simulink model "Super3"  (Simulink 5.0)
settings: Solver=ode45  StartTime=0.0  StopTime=10.0  RelTol=1e-3
undefined symbols (not defined in the file): sigbuilder_block
settings Model: Creator=scaife  LastModifiedBy=scaife  ExtModeAutoUpdateStatusClock=off

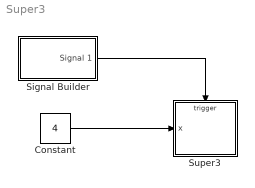
== system Super3 ==
  Constant : Constant  Value=4
  Signal Builder : Subsystem  Tag=STV Subsys  StartFcn=sigbuilder_block('start');  StopFcn=sigbuilder_block('stop');  ClipboardFcn=sigbuilder_block('clipboard');  mask(Sigbuilder block){}
      mask help: Sigbuilder GUI
      mask init:
      | if ~strcmp(get_param(bdroot(gcb),'SimulationStatus'),'stopped') tuvar = sigbuilder_block('maskInit'); end
      settings: CopyFcn=sigbuilder_block('copy');  DeleteFcn=sigbuilder_block('delete');  ModelCloseFcn=sigbuilder_block('modelClose');  PreSaveFcn=sigbuilder_block('preSave');  NameChangeFcn=sigbuilder_block('namechange');  OpenFcn=sigbuilder_block('open',[50 50 520 400 ]);  CloseFcn=sigbuilder_block('close');
      mask Display: plot(0,0,100,100,[10,10,40,40,10],[80,20,20,80,80],[40,10],[50,50], [40,27,10],[65,72,56],[40,25,25,10],[28,28,43,43]);
  Super3 : Stateflow chart
  wires:
  Signal Builder/1(Signal 1) -> Super3/Trigger
  Constant/1 -> Super3/1(x)

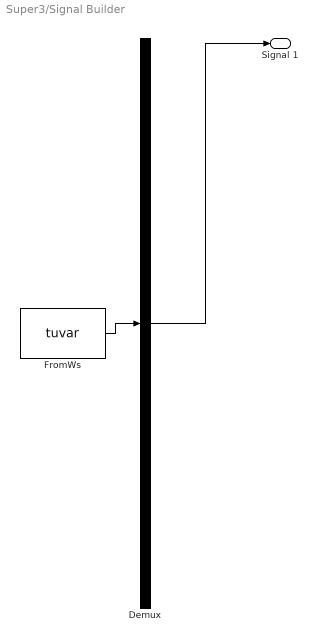
== system Super3/Signal Builder ==
  Demux : Demux  Tag=STV Demux  Outputs=1
  FromWs : FromWorkspace  Tag=STV FromWs  VariableName=tuvar  SampleTime=0  SigBuilderData=DataTag0
  Signal 1 : Outport  Tag=STV Outport
  wires:
  Demux/1 -> Signal 1/1
  FromWs/1 -> Demux/1

== stateflow chart Super3 ==
  state A
  state C
  state B
    state B1
    state B2
    B1 -> (junction 10) : E[x>3]
    (junction 10) -> B2 : [x==4]
    (default) -> B1
    (junction 11) -> B2 : E[x==3]
    B1 -> (junction 11) : E[x<=3]
    B2 -> B : E[x==3||x==4]
  state D
  A -> (junction 9) : E
  (junction 9) -> B1 : [x>0]
  (junction 9) -> D : [x==0]
  D -> B : E[x==0]
  (default) -> A
  (junction 10) -> C : [x==5]
  B -> C : E[x==0]
  B1 -> A : E[x==2]
  (junction 11) -> D : E[x==1]
  C -> A : E[x==0||x==5]
  D -> A : E[x==1]
  data: x input int32
  events: E input EITHER_EDGE_EVENT
